simulink model "pid1111"  (R2023a)
settings: Solver=FixedStepAuto  StartTime=0.0  StopTime=300  FixedStep=0.0001  RelTol=1e-3
model workspace (MAT data in the model file):
  t = Simulink.Parameter
  t.DataType = 'auto'
  t.Complexity = 'real'
  t.Dimensions = [0 0]
values from neighbouring files (symbols this model uses):
  A1 = [0 1 0 0 ... (first row only)    [pid1111.m]
  A2 = [0 1 ... (first row only)    [pid1111.m]
  amp = 0.01    [MS_PID_Test.m]    (also in pid1111.m)
  B1 = [0 k_m/m2 0 -k_m/m2]'    [pid1111.m]
  B2 = 0    [pid1111.m]
  C1 = [-k1/m1 -c1/m1 k1/m1 c1/m1 ... (first row only)    [pid1111.m]
  C2 = [1 0]    [pid1111.m]
  D1 = 0    [pid1111.m]
  D2 = 0    [pid1111.m]
  E1 = [0 0 0 c2/m2 ... (first row only)    [pid1111.m]
  E2 = [0 0 ... (first row only)    [pid1111.m]
  fre = 31.3    [pid1111.m]
  Kd = 00070    (= 70)    [MS_PID_Test.m]    (also in paper_repro.m = 0.1; pid1111.m)
  Ki = 13000    [MS_PID_Test.m]    (also in paper_repro.m = 1; pid1111.m)
  Kp = 27000    [MS_PID_Test.m]    (also in paper_repro.m = 10000; pid1111.m)
libraries: slpidlib x1
settings Model: Creator=z'k'x  LastModifiedBy=z'k'x

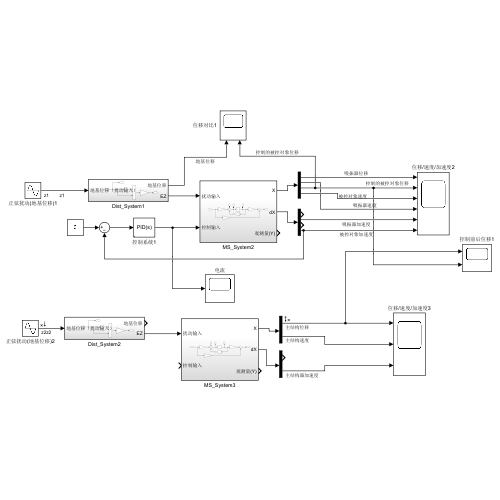
[thumbnail: Simulink's stored preview of the top-level diagram]
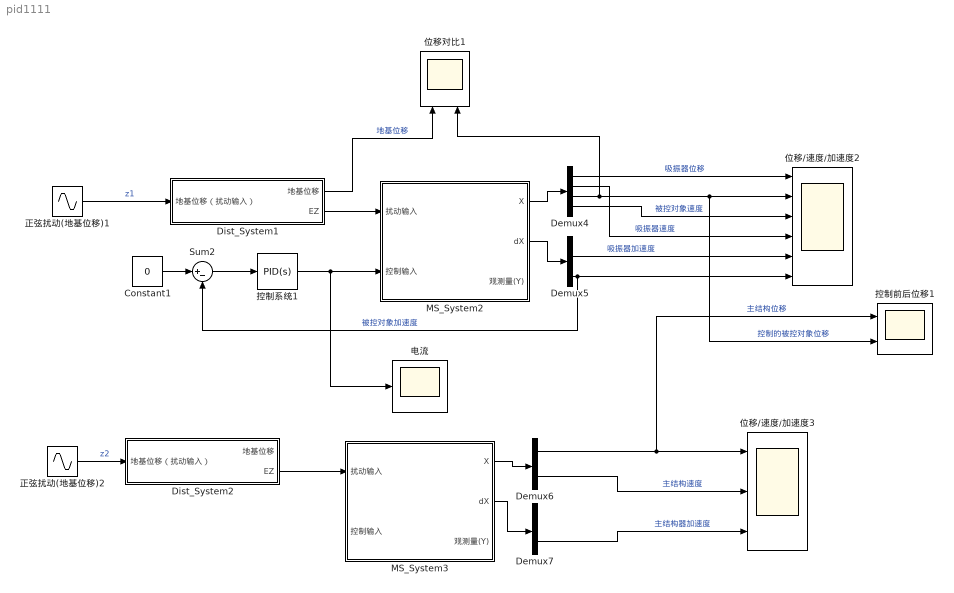
== system pid1111 ==
  Constant1 : Constant  Value=0
  Demux4 : Demux
  Demux5 : Demux
  Demux6 : Demux  Outputs=2
  Demux7 : Demux  Outputs=2
  Dist_System1 : Subsystem
  Dist_System2 : Subsystem
  MS_System2 : Subsystem
  MS_System3 : Subsystem
  Sum2 : Sum  Inputs=|+-
  位移/速度/加速度2 : Scope  NumInputPorts=6
  位移/速度/加速度3 : Scope  NumInputPorts=3
  位移对比1 : Scope  NumInputPorts=2
  控制前后位移1 : Scope  NumInputPorts=2
  控制系统1 : slpidlib/PID Controller  Controller=PID  Form=Parallel  TimeDomain=Continuous-time  UseExternalTs=off  SampleTime=-1  IntegratorMethod=Forward Euler  FilterMethod=Forward Euler  ControllerParametersSource=internal  P=Kp  I=Ki  UseKiTs=off  D=Kd  N=100  UseFilter=on  TunerSelectOption=Transfer Function Based (PID Tuner App)  InitialConditionSource=internal  InitialConditionForIntegrator=0  InitialConditionForFilter=0  DifferentiatorICPrevScaledInput=0  ExternalReset=none  TrackingMode=off  Kt=1  LimitOutput=off  SatLimitsSource=internal  UpperSaturationLimit=inf  LowerSaturationLimit=-inf  LinearizeAsGain=on  AntiWindupMode=none  Kb=1  LimitIntegrator=off  UpperIntegratorSaturationLimit=inf  LowerIntegratorSaturationLimit=-inf  POutMin=[]  POutMax=[]  IOutMin=[]  IOutMax=[]  DOutMin=[]  DOutMax=[]  NOutMin=[]  NOutMax=[]  SumOutMin=[]  SumOutMax=[]  SaturationOutMin=[]  SaturationOutMax=[]  PParamMin=[]  PParamMax=[]  IParamMin=[]  IParamMax=[]  DParamMin=[]  DParamMax=[]  NParamMin=[]  NParamMax=[]  KbParamMin=[]  KbParamMax=[]  KtParamMin=[]  KtParamMax=[]  KbOutMin=[]  KbOutMax=[]  KtOutMin=[]  KtOutMax=[]  IntegratorOutMin=[]  IntegratorOutMax=[]  FilterOutMin=[]  FilterOutMax=[]  SumI1OutMin=[]  SumI1OutMax=[]  SumI2OutMin=[]  SumI2OutMax=[]  SumI3OutMin=[]  SumI3OutMax=[]  SumI4OutMin=[]  SumI4OutMax=[]  SumDOutMin=[]  SumDOutMax=[]  DifferentiatorOutMin=[]  DifferentiatorOutMax=[]  FilterDiffOutCoefMin=[]  FilterDiffOutCoefMax=[]  ReciprocalOutMin=[]  ReciprocalOutMax=[]  SumDenOutMin=[]  SumDenOutMax=[]  SumNumOutMin=[]  SumNumOutMax=[]  DivideOutMin=[]  DivideOutMax=[]  UdiffTsProdOutMin=[]  UdiffTsProdOutMax=[]  NTsProdOutMin=[]  NTsProdOutMax=[]  UintegralTsProdOutMin=[]  UintegralTsProdOutMax=[]  UngainTsProdOutMin=[]  UngainTsProdOutMax=[]  ClampingZeroOutDataTypeStr=Inherit: Inherit via back propagation  ClampingZeroOutMin=[]  ClampingZeroOutMax=[]  FilterDenConstantOutDataTypeStr=Inherit: Inherit via back propagation  FilterDenConstantOutMin=[]  FilterDenConstantOutMax=[]  PCopyOutDataTypeStr=Inherit: Inherit via back propagation  PCopyOutMin=[]  PCopyOutMax=[]  NCopyOutDataTypeStr=Inherit: Inherit via back propagation  NCopyOutMin=[]  NCopyOutMax=[]  IntegratorContinuousStateAttributes=''  IntegratorStateMustResolveToSignalObject=off  IntegratorRTWStateStorageClass=Auto  FilterContinuousStateAttributes=''  FilterStateMustResolveToSignalObject=off  FilterRTWStateStorageClass=Auto  ParallelPVariant=InternalParameters  IdealPVariant=Disabled  IVariant=InternalParameters  DVariant=InternalParameters  IntegratorVariant=Continuous  SatVariant=Disabled  AWVariant=Passthrough  PCopyVariant=Disabled  TRVariant=Disabled  FdbkBlocksVariant=Forward  IdealPFdbkVariant=Disabled  SatFdbkVariant=Disabled  DerivativeFilterVariant=ContFilter  NVariant=InternalParameters  NCopyVariant=Disabled  FilterICVariant=InternalICsFilter  IntegratorICVariant=InternalICs  ExternalResetVariant=Disabled  TRSumVariant=Passthrough  SumFdbkVariant=Disabled  SumVariant=Sum_PID  TsampFilterVariant=InternalTs  TsampNgainVariant=Passthrough  TsampIntegralVariant=Disabled_SignalSpec  ExternalSaturationOutDataTypeStr=Inherit: Same as second input
  正弦扰动(地基位移)1 : Sin  Amplitude=amp  Frequency=fre  SampleTime=0
  正弦扰动(地基位移)2 : Sin  Amplitude=amp  Frequency=fre  SampleTime=0
  电流 : Scope
  wires:
  控制系统1/1 -> MS_System2/2(控制输入), 电流/1
  Demux6/2 -> 位移/速度/加速度3/2  "主结构速度"
  Dist_System1/2(EZ) -> MS_System2/1(扰动输入)
  MS_System3/2(dX) -> Demux7/1
  正弦扰动(地基位移)1/1 -> Dist_System1/1(地基位移（扰动输入）)  "z1"
  MS_System2/1(X) -> Demux4/1
  Demux7/2 -> 位移/速度/加速度3/3  "主结构器加速度"
  Demux5/2 -> 位移/速度/加速度2/5  "吸振器加速度"
  Demux4/1 -> 位移/速度/加速度2/1  "吸振器位移"
  Demux4/4 -> 位移/速度/加速度2/3  "被控对象速度"
  Constant1/1 -> Sum2/1
  Dist_System1/1(地基位移) -> 位移对比1/1  "地基位移"
  Demux4/3 -> 位移对比1/2, 控制前后位移1/2, 位移/速度/加速度2/2  "控制的被控对象位移"
  MS_System2/2(dX) -> Demux5/1
  Sum2/1 -> 控制系统1/1
  Demux4/2 -> 位移/速度/加速度2/4  "吸振器速度"
  正弦扰动(地基位移)2/1 -> Dist_System2/1(地基位移（扰动输入）)  "z2"
  Demux5/4 -> Sum2/2, 位移/速度/加速度2/6  "被控对象加速度"
  MS_System3/1(X) -> Demux6/1
  Demux6/1 -> 位移/速度/加速度3/1, 控制前后位移1/1  "主结构位移"
  Dist_System2/2(EZ) -> MS_System3/1(扰动输入)

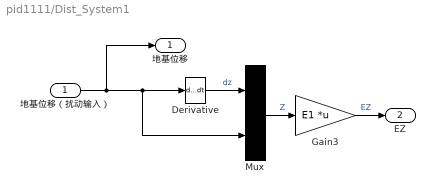
== system pid1111/Dist_System1 ==
  地基位移（扰动输入） : Inport
  Derivative : Derivative
  Gain3 : Gain  Gain=E1  Multiplication=Matrix(K*u) (u vector)
  Mux : Mux  Inputs=2
      settings: DisplayOption=signals
  地基位移 : Outport
  EZ : Outport  Port=2
  wires:
  Gain3/1 -> EZ/1  "EZ"
  Mux/1 -> Gain3/1  "Z"
  Derivative/1 -> Mux/1  "dz"
  地基位移（扰动输入）/1 -> 地基位移/1, Derivative/1, Mux/2

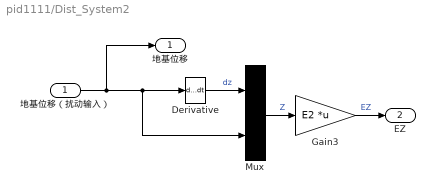
== system pid1111/Dist_System2 ==
  地基位移（扰动输入） : Inport
  Derivative : Derivative
  Gain3 : Gain  Gain=E2  Multiplication=Matrix(K*u) (u vector)
  Mux : Mux  Inputs=2
      settings: DisplayOption=signals
  地基位移 : Outport
  EZ : Outport  Port=2
  wires:
  Gain3/1 -> EZ/1  "EZ"
  Mux/1 -> Gain3/1  "Z"
  Derivative/1 -> Mux/1  "dz"
  地基位移（扰动输入）/1 -> 地基位移/1, Derivative/1, Mux/2

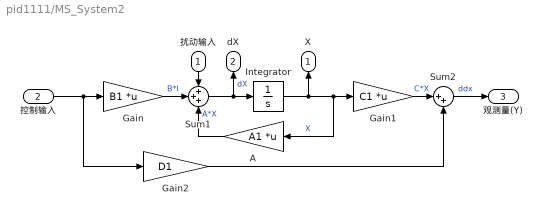
== system pid1111/MS_System2 ==
  扰动输入 : Inport
  控制输入 : Inport  Port=2
  A : Gain  Gain=A1  Multiplication=Matrix(K*u) (u vector)
  Gain : Gain  Gain=B1  Multiplication=Matrix(K*u) (u vector)
  Gain1 : Gain  Gain=C1  Multiplication=Matrix(K*u) (u vector)
  Gain2 : Gain  Gain=D1
  Integrator : Integrator
  Sum1 : Sum  Inputs=+++
  Sum2 : Sum  Inputs=|++
  X : Outport
  dX : Outport  Port=2
  观测量(Y) : Outport  Port=3
  wires:
  Gain2/1 -> Sum2/2
  Integrator/1 -> A/1, Gain1/1, X/1  "X"
  Sum1/1 -> dX/1, Integrator/1  "dX"
  Gain/1 -> Sum1/2  "B*I"
  Gain1/1 -> Sum2/1  "C*X"
  A/1 -> Sum1/3  "A*X"
  Sum2/1 -> 观测量(Y)/1  "ddx"
  控制输入/1 -> Gain2/1, Gain/1
  扰动输入/1 -> Sum1/1

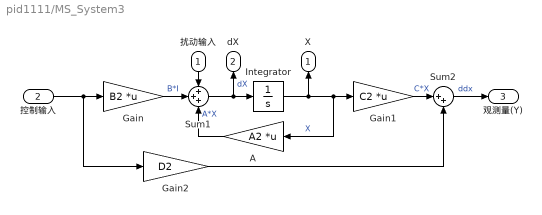
== system pid1111/MS_System3 ==
  扰动输入 : Inport
  控制输入 : Inport  Port=2
  A : Gain  Gain=A2  Multiplication=Matrix(K*u) (u vector)
  Gain : Gain  Gain=B2  Multiplication=Matrix(K*u) (u vector)
  Gain1 : Gain  Gain=C2  Multiplication=Matrix(K*u) (u vector)
  Gain2 : Gain  Gain=D2
  Integrator : Integrator
  Sum1 : Sum  Inputs=+++
  Sum2 : Sum  Inputs=|++
  X : Outport
  dX : Outport  Port=2
  观测量(Y) : Outport  Port=3
  wires:
  Gain2/1 -> Sum2/2
  Integrator/1 -> A/1, Gain1/1, X/1  "X"
  Sum1/1 -> dX/1, Integrator/1  "dX"
  Gain/1 -> Sum1/2  "B*I"
  Gain1/1 -> Sum2/1  "C*X"
  A/1 -> Sum1/3  "A*X"
  Sum2/1 -> 观测量(Y)/1  "ddx"
  控制输入/1 -> Gain2/1, Gain/1
  扰动输入/1 -> Sum1/1
